simulink model "model2"  (R2024a)
settings: Solver=VariableStepAuto  StartTime=0.0  StopTime=10  MaxStep=1e-5  RelTol=1e-5
values from neighbouring files (symbols this model uses):
  A = [8 1 11 ... (first row only)    [init.m]
  A_bar = [G_f,          zero_1 ... (first row only)    [init.m]
  B = [-1; -3; 3]    [init.m]
  B_bar = [zeros(r, size(B, 2)) ... (first row only)    [init.m]
  B_f = [1, -1 ... (first row only)    [init.m]
  C = [-2 0 -3]    [init.m]
  C_bar = [D_f * Y_f, C]    [init.m]
  D = 15    [init.m]
  D_f = [0 3]    [init.m]
  G = [-5 0 0 ... (first row only)    [init.m]
  G_f = [35 10 -28 17 ... (first row only)    [init.m]
  G_g = [0 0 0 ... (first row only)    [init.m]
  K = [-3.5 1 -3.5]    [init.m]
  K_f = [-9.2262   -2.9556    6.9958   -4.9150]    [init.m]
  K_g = [0.0703   -0.0562    0.0658]    [init.m]
  L = 2.5    [init.m]
  Q_inv = pinv(Q)    [init.m]
  wf0 = [1; 1; 1; 1]    [init.m]
  wg0 = [-12; 0; 21]    [init.m]
  x0 = [0; 0; 0]    [init.m]
  Y = [1; 7; 8]    [init.m]
  Y_f = [12 -6 ... (first row only)    [init.m]
  Y_g = [1, 1, 0]    [init.m]
settings Model: Creator=eva  LastModifiedBy=eva

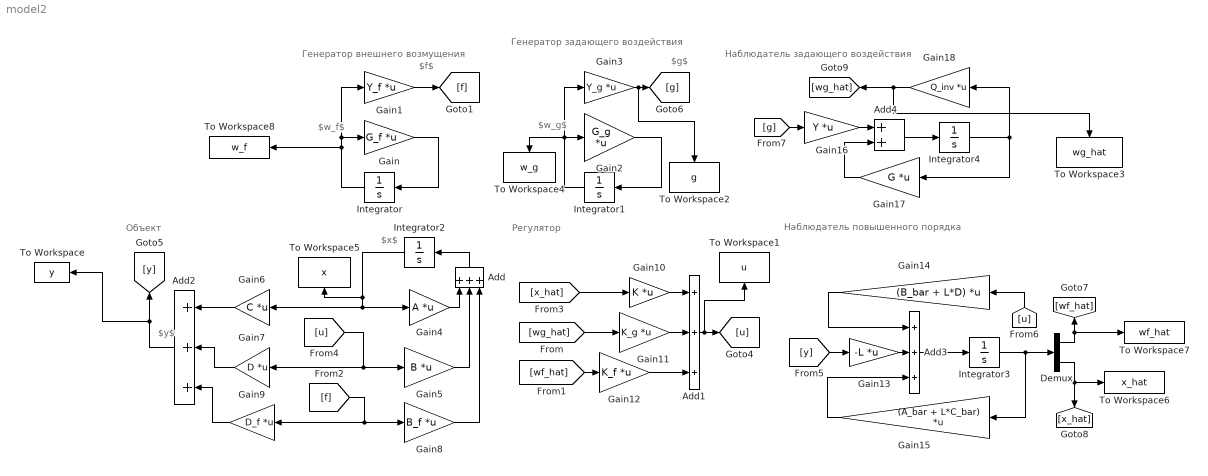
== system model2 ==
  note: Наблюдатель повышенного порядка
  note: Наблюдатель задающего воздействия
  note: Генератор внешнего возмущения
  note: Объект
  note: Регулятор
  note: $g$
  note: $w_f$
  note: Генератор задающего воздействия
  note: $x$
  note: $y$
  note: $w_g$
  note: $f$
  Add{,1..3} (4 alike) : Sum  Inputs=+++
  Add4 : Sum
  Demux : Demux  Outputs=2
  Gain : Gain  Gain=G_f  Multiplication=Matrix(K*u)
  Gain1 : Gain  Gain=Y_f  Multiplication=Matrix(K*u)
  Gain10 : Gain  Gain=K  Multiplication=Matrix(K*u)
  Gain11 : Gain  Gain=K_g  Multiplication=Matrix(K*u)
  Gain12 : Gain  Gain=K_f  Multiplication=Matrix(K*u)
  Gain13 : Gain  Gain=-L  Multiplication=Matrix(K*u)
  Gain14 : Gain  Gain=(B_bar + L*D)  Multiplication=Matrix(K*u)
  Gain15 : Gain  Gain=(A_bar + L*C_bar)  Multiplication=Matrix(K*u)
  Gain16 : Gain  Gain=Y  Multiplication=Matrix(K*u)
  Gain17 : Gain  Gain=G  Multiplication=Matrix(K*u)
  Gain18 : Gain  Gain=Q_inv  Multiplication=Matrix(K*u)
  Gain2 : Gain  Gain=G_g  Multiplication=Matrix(K*u)
  Gain3 : Gain  Gain=Y_g  Multiplication=Matrix(K*u)
  Gain4 : Gain  Gain=A  Multiplication=Matrix(K*u)
  Gain5 : Gain  Gain=B  Multiplication=Matrix(K*u)
  Gain6 : Gain  Gain=C  Multiplication=Matrix(K*u)
  Gain7 : Gain  Gain=D  Multiplication=Matrix(K*u)
  Gain8 : Gain  Gain=B_f  Multiplication=Matrix(K*u)
  Gain9 : Gain  Gain=D_f  Multiplication=Matrix(K*u)
  Integrator : Integrator  InitialCondition=wf0
  Integrator1 : Integrator  InitialCondition=wg0
  Integrator2 : Integrator  InitialCondition=x0
  Integrator3 : Integrator
  Integrator4 : Integrator
  To Workspace : ToWorkspace  VariableName=y  SaveFormat=Structure With Time  SampleTime=-1
  To Workspace1 : ToWorkspace  VariableName=u  SaveFormat=Structure With Time  SampleTime=-1
  To Workspace2 : ToWorkspace  VariableName=g  SaveFormat=Structure With Time  SampleTime=-1
  To Workspace3 : ToWorkspace  VariableName=wg_hat  SaveFormat=Structure With Time  SampleTime=-1
  To Workspace4 : ToWorkspace  VariableName=w_g  SaveFormat=Structure With Time  SampleTime=-1
  To Workspace5 : ToWorkspace  VariableName=x  SaveFormat=Structure With Time  SampleTime=-1
  To Workspace6 : ToWorkspace  VariableName=x_hat  SaveFormat=Structure With Time  SampleTime=-1
  To Workspace7 : ToWorkspace  VariableName=wf_hat  SaveFormat=Structure With Time  SampleTime=-1
  To Workspace8 : ToWorkspace  VariableName=w_f  SaveFormat=Structure With Time  SampleTime=-1
  wires:
  Gain11/1 -> Add1/2
  Integrator/1 -> To Workspace8/1, Gain/1, Gain1/1
  Add/1 -> Integrator2/1
  Gain/1 -> Integrator/1
  [u] -> Gain7/1, Gain5/1
  [wf_hat] -> Gain12/1
  Gain2/1 -> Integrator1/1
  Gain10/1 -> Add1/1
  Gain1/1 -> [f]
  Gain5/1 -> Add/2
  Gain6/1 -> Add2/1
  [x_hat] -> Gain10/1
  Integrator1/1 -> To Workspace4/1, Gain2/1, Gain3/1
  Add1/1 -> To Workspace1/1, [u]
  [wg_hat] -> Gain11/1
  [f] -> Gain8/1, Gain9/1
  Gain8/1 -> Add/3
  Add2/1 -> To Workspace/1, [y]
  Integrator2/1 -> Gain6/1, Gain4/1, To Workspace5/1
  Gain12/1 -> Add1/3
  Gain4/1 -> Add/1
  Gain7/1 -> Add2/2
  Gain3/1 -> To Workspace2/1, [g]
  Gain9/1 -> Add2/3
  [y] -> Gain13/1
  [u] -> Gain14/1
  Add3/1 -> Integrator3/1
  Integrator3/1 -> Gain15/1, Demux/1
  Gain15/1 -> Add3/3
  Demux/1 -> To Workspace7/1, [wf_hat]
  Demux/2 -> To Workspace6/1, [x_hat]
  Gain16/1 -> Add4/1
  Add4/1 -> Integrator4/1
  Integrator4/1 -> Gain17/1, Gain18/1
  Gain17/1 -> Add4/2
  Gain18/1 -> To Workspace3/1, [wg_hat]
  Gain13/1 -> Add3/2
  Gain14/1 -> Add3/1
  [g] -> Gain16/1
